simulink model "without_treatment"  (R2021b)
settings: Solver=VariableStepAuto  StartTime=0.0  StopTime=90000  RelTol=1e-3
settings Model: Creator=Rasoul  LastModifiedBy=Rasoul

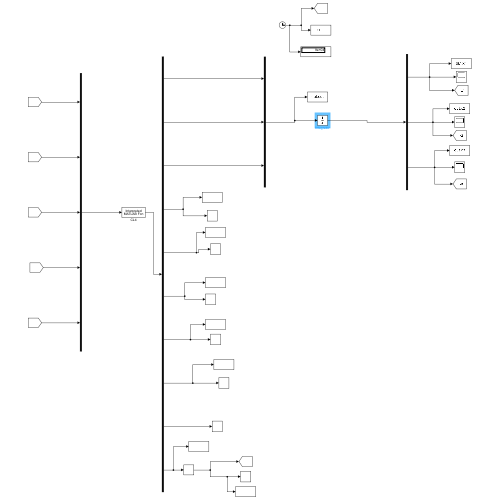
[thumbnail: Simulink's stored preview of the top-level diagram]
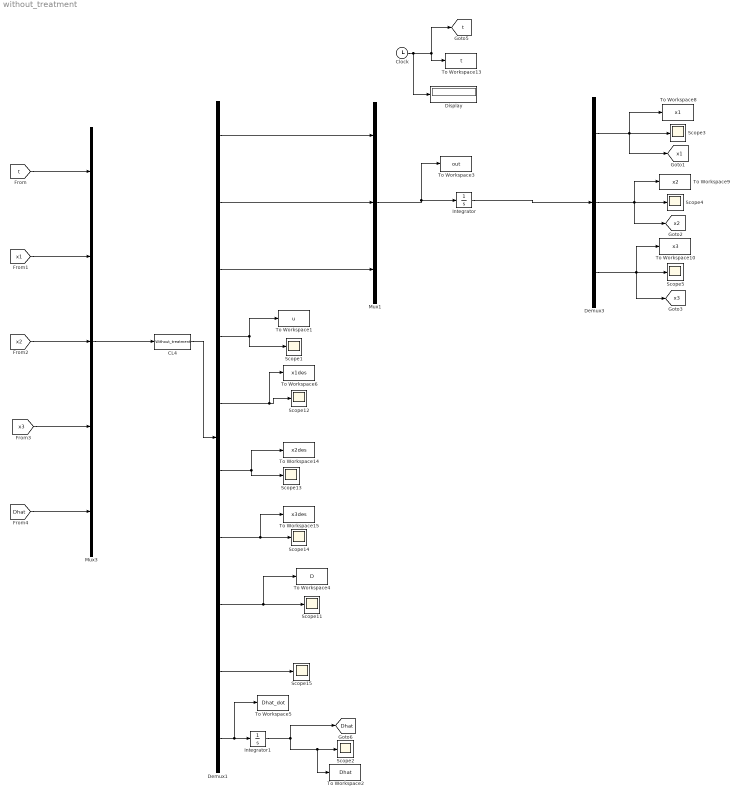
== system without_treatment ==
  CL4 : MATLABFcn  MATLABFcn=Without_treatment  OutputDimensions=10
  Clock : Clock
  Demux1 : Demux  Outputs=10
  Demux3 : Demux  Outputs=3
  Display : Display
  Integrator : Integrator  InitialCondition=[150;0;100]
  Integrator1 : Integrator
  Mux1 : Mux  Inputs=3
  Mux3 : Mux  Inputs=5
  Scope{1..5,11..15} (10 alike) : Scope
  To Workspace1 : ToWorkspace  VariableName=u  SampleTime=10
      settings: Save2DSignal=2-D array (concatenate along first dimension)
  To Workspace10 : ToWorkspace  VariableName=x3  SampleTime=10
      settings: Save2DSignal=2-D array (concatenate along first dimension)
  To Workspace13 : ToWorkspace  VariableName=t  SampleTime=10
      settings: Save2DSignal=2-D array (concatenate along first dimension)
  To Workspace14 : ToWorkspace  VariableName=x2des  SampleTime=10
      settings: Save2DSignal=2-D array (concatenate along first dimension)
  To Workspace15 : ToWorkspace  VariableName=x3des  SampleTime=10
      settings: Save2DSignal=2-D array (concatenate along first dimension)
  To Workspace2 : ToWorkspace  VariableName=Dhat  SampleTime=10
      settings: Save2DSignal=2-D array (concatenate along first dimension)
  To Workspace3 : ToWorkspace  VariableName=out  SampleTime=-1
      settings: Save2DSignal=2-D array (concatenate along first dimension)
  To Workspace4 : ToWorkspace  VariableName=D  SampleTime=10
      settings: Save2DSignal=2-D array (concatenate along first dimension)
  To Workspace5 : ToWorkspace  VariableName=Dhat_dot  SampleTime=10
      settings: Save2DSignal=2-D array (concatenate along first dimension)
  To Workspace6 : ToWorkspace  VariableName=x1des  SampleTime=10
      settings: Save2DSignal=2-D array (concatenate along first dimension)
  To Workspace8 : ToWorkspace  VariableName=x1  SampleTime=10
      settings: Save2DSignal=2-D array (concatenate along first dimension)
  To Workspace9 : ToWorkspace  VariableName=x2  SampleTime=10
      settings: Save2DSignal=2-D array (concatenate along first dimension)
  tag scope: Dhat=global, t=global, x1=global, x2=global, x3=global
  wires:
  Clock/1 -> Display/1, [t], To Workspace13/1
  Integrator1/1 -> To Workspace2/1, Scope2/1, [Dhat]
  Demux1/2 -> Mux1/2
  Mux1/1 -> To Workspace3/1, Integrator/1
  [Dhat] -> Mux3/5
  Demux1/5 -> Scope12/1, To Workspace6/1
  Integrator/1 -> Demux3/1
  Demux1/9 -> Scope15/1
  CL4/1 -> Demux1/1
  Demux1/8 -> To Workspace4/1, Scope11/1
  Demux1/4 -> To Workspace1/1, Scope1/1
  Demux1/6 -> To Workspace14/1, Scope13/1
  Demux1/3 -> Mux1/3
  Demux1/10 -> To Workspace5/1, Integrator1/1
  [x2] -> Mux3/3
  Demux1/1 -> Mux1/1
  [t] -> Mux3/1
  Demux1/7 -> To Workspace15/1, Scope14/1
  Mux3/1 -> CL4/1
  [x1] -> Mux3/2
  Demux3/2 -> To Workspace9/1, Scope4/1, [x2]
  Demux3/3 -> To Workspace10/1, Scope5/1, [x3]
  [x3] -> Mux3/4
  Demux3/1 -> To Workspace8/1, Scope3/1, [x1]
